simulink model "NUOVO_MODELLO_COPPIE_VELOCITA"  (R2021a)
settings: Solver=VariableStepAuto  StartTime=0.0  StopTime=3  RelTol=1e-3
values from neighbouring files (symbols this model uses):
  A = [1 Ts;0 1]    [parameters.m]
  Be = 1    [parameters.m]
  beta = 2*pi*Fc*Ts / (1+2*pi*Fc*Ts)    (= 0.00624395339097)    [parameters.m]
  Bh = 0.002    [parameters.m]
  Bh_hat = 0.0002    [parameters.m]
  C = [1 0]    [parameters.m]
  delayCommM2S = 0    [parameters.m]
  delayCommS2M = 0    [parameters.m]
  dt = 0.5    [parameters.m]
  Fc = 1    [parameters.m]
  Jh = 0.00002    (= 2e-05)    [parameters.m]
  k_m = 19.34    [parameters.m]
  k_s = 19.34    [parameters.m]
  Kc2v_m = 2    [parameters.m]
  Kc2v_s = 2    [parameters.m]
  Kd_h = 1.125    [parameters.m]
  Ke = 10    [parameters.m]
  Kh_hat = 0.0002    [parameters.m]
  Kh_max = 50    [parameters.m]
  Kp_h = 0.8    [parameters.m]
  Kt2c_m = 1.182    [parameters.m]
  Kt2c_s = 1.182    [parameters.m]
  lArm_m = 0.1    [parameters.m]
  lArm_s = 0.1    [parameters.m]
  noise_threshold = 0.05    [parameters.m]
  PosRef = 1    [parameters.m]
  qe = 2    [parameters.m]
  stopTime = str2double(stopTime)    [parameters.m]
  tau_m = 1.217    [parameters.m]
  tau_s = 1.217    [parameters.m]
  Ts = 0.001    [parameters.m]
  Variance = 0.00000001    (= 1e-08)    [parameters.m]
undefined symbols (not defined in the file or in its folder): DiscIntNeverNeededParam, Discrete, Time
libraries: simulink_extras x20, dspsigops x20, ctrlSharedLib x7, cstblocks x1
settings Model: Creator=mirko  LastModifiedBy=mirko

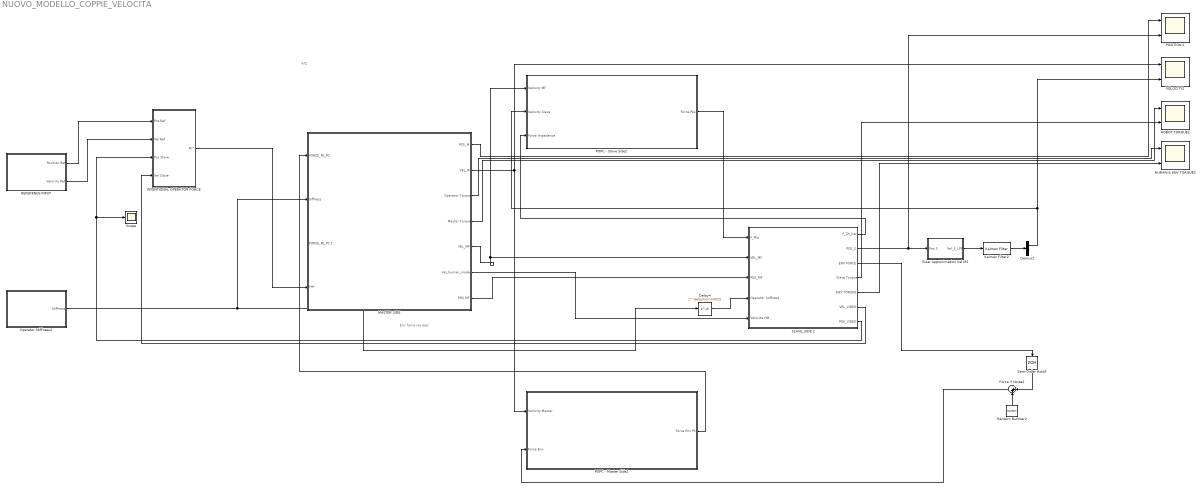
== system NUOVO_MODELLO_COPPIE_VELOCITA ==
  note: A/Z
  note: Env force revised
  Delay4 : Delay  DelayLength=delayCommM2S  SampleTime=Ts
  Demux2 : Demux  Outputs=2
  Euler Approximation Vel M2 : Subsystem
  Force + Noise2 : Sum  Inputs=|++
  HUMAN & ENV TORQUE2 : Scope  NumInputPorts=2
  INTENTIONAL OPERATOR FORCE : Subsystem
  Kalman Filter2 : ctrlSharedLib/Kalman Filter  TimeDomain=Discrete-Time  UseCurrentEstimator=off  ModelSource=Individual A, B, C, D matrices  ModelSourceVariable=ss(A,0,C,0)  A=A  B=1  C=C  D=0  NumberOfStates=2  NumberOfInputs=1  NumberOfOutputs=1  InitialEstimateSource=Dialog  X0=0  P0=10  UseK=off  UseGH=off  NumberOfProcessNoiseInputs=1  G=1  TimeInvariantG=on  H=0  TimeInvariantH=on  Q=0.05  TimeInvariantQ=on  R=1  TimeInvariantR=on  N=0  TimeInvariantN=on  AddInputPort=off  AddEnablePort=off  OutputEstimatedY=off  OutputP=off  Ts=Ts
  MASTER SIDE : Subsystem
  Operator Stiffness2 : Subsystem
  POPC - Master Side2 : Subsystem
  POPC - Slave Side2 : Subsystem
  POSITION 2 : Scope  NumInputPorts=2
  REFERENCE INPUT : Subsystem
  ROBOT TORQUE2 : Scope  NumInputPorts=2
  Random Number2 : RandomNumber  Variance=Variance  SampleTime=Ts
  SLAVE_SIDE 2 : Subsystem
  Scope : Scope
  VELOCITY2 : Scope  NumInputPorts=2
  Zero-Order Hold3 : ZeroOrderHold  SampleTime=Ts
  wires:
  Operator Stiffness2/1(Stiffness) -> Delay4/1, MASTER SIDE/2(Siffness)
  Force + Noise2/1 -> POPC - Master Side2/2(Force Env)
  REFERENCE INPUT/2("Velocity Ref ") -> INTENTIONAL OPERATOR FORCE/2(Vel Ref)
  POPC - Slave Side2/1(Force PCs) -> SLAVE_SIDE 2/1(F_PCs)
  Demux2/1 -> VELOCITY2/2, POPC - Slave Side2/2(Velocity Slave)
  SLAVE_SIDE 2/1(F_Zh_hat) -> POPC - Slave Side2/3(Force Impedence)
  MASTER SIDE/4(Master Torque) -> ROBOT TORQUE2/1
  Random Number2/1 -> Force + Noise2/2
  MASTER SIDE/3(Operator Torque) -> HUMAN & ENV TORQUE2/1
  SLAVE_SIDE 2/2(POS_S) -> POSITION 2/2, Euler Approximation Vel M2/1(Pos S)
  REFERENCE INPUT/1("Position Ref ") -> INTENTIONAL OPERATOR FORCE/1(Pos Ref)
  POPC - Master Side2/1(Force Env PC) -> MASTER SIDE/1("FORCE_FE_PC ")
  SLAVE_SIDE 2/7(POS_VIDEO) -> INTENTIONAL OPERATOR FORCE/3(Pos Slave), Scope/1
  SLAVE_SIDE 2/3(ENV FORCE) -> Zero-Order Hold3/1
  SLAVE_SIDE 2/5(ENV TORQUE) -> HUMAN & ENV TORQUE2/2
  SLAVE_SIDE 2/6(VEL_VIDEO) -> INTENTIONAL OPERATOR FORCE/4(Vel Slave)
  MASTER SIDE/2(VEL_M) -> POPC - Master Side2/1(Velocity Master), VELOCITY2/1
  Kalman Filter2/1 -> Demux2/1
  Delay4/1 -> SLAVE_SIDE 2/4(Operator Stiffness)
  Zero-Order Hold3/1 -> Force + Noise2/1
  Euler Approximation Vel M2/1("Vel_S_LPF ") -> Kalman Filter2/1
  SLAVE_SIDE 2/4(Slave Torque) -> ROBOT TORQUE2/2
  MASTER SIDE/1(POS_M) -> POSITION 2/1
  INTENTIONAL OPERATOR FORCE/1("Fh* ") -> MASTER SIDE/4(FH*)
  MASTER SIDE/5(VEL_MF) -> POPC - Slave Side2/1(Velocity MF), SLAVE_SIDE 2/2(VEL_MF)
  MASTER SIDE/6(Vel_human_model) -> SLAVE_SIDE 2/5("Velocità HM ")
  MASTER SIDE/7(POS MF) -> SLAVE_SIDE 2/3(POS_MF)

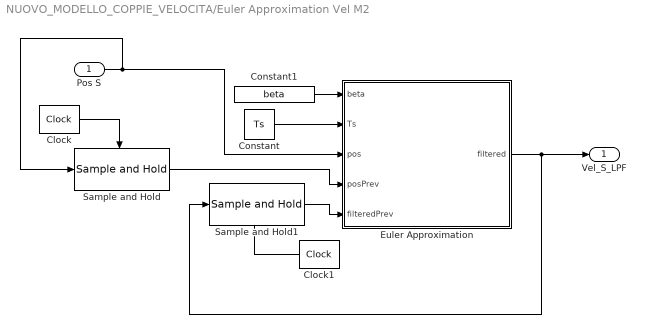
== system NUOVO_MODELLO_COPPIE_VELOCITA/Euler Approximation Vel M2 ==
  Pos S : Inport
  Clock : simulink_extras/Flip Flops/Clock  period=Ts*2
  Clock1 : simulink_extras/Flip Flops/Clock  period=Ts*2
  Constant : Constant  Value=Ts
  Constant1 : Constant  Value=beta
  "Euler Approximation " : MATLAB Function  TreatAsAtomicUnit=on
  Sample and Hold : dspsigops/Sample and Hold  trig=Rising edge  initCond=0  latchinput=on
  Sample and Hold1 : dspsigops/Sample and Hold  trig=Rising edge  initCond=0  latchinput=on
  "Vel_S_LPF " : Outport
  wires:
  Pos S/1 -> Sample and Hold/1, "Euler Approximation "/3(pos)
  Constant/1 -> "Euler Approximation "/2(Ts)
  Sample and Hold/1 -> "Euler Approximation "/4(posPrev)
  Clock/1 -> Sample and Hold/Trigger
  Sample and Hold1/1 -> "Euler Approximation "/5(filteredPrev)
  "Euler Approximation "/1(filtered) -> "Vel_S_LPF "/1, Sample and Hold1/1
  Clock1/1 -> Sample and Hold1/Trigger
  Constant1/1 -> "Euler Approximation "/1(beta)

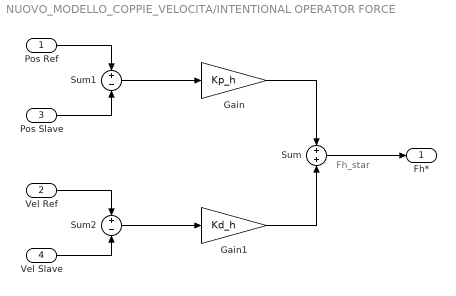
== system NUOVO_MODELLO_COPPIE_VELOCITA/INTENTIONAL OPERATOR FORCE ==
  note: Fh_star
  Pos Ref : Inport
  Vel Ref : Inport  Port=2
  Pos Slave : Inport  Port=3
  Vel Slave : Inport  Port=4
  Gain : Gain  Gain=Kp_h
  Gain1 : Gain  Gain=Kd_h
  Sum : Sum
  Sum1 : Sum  Inputs=+-
  Sum2 : Sum  Inputs=+-
  "Fh* " : Outport
  wires:
  Pos Ref/1 -> Sum1/1
  Pos Slave/1 -> Sum1/2
  Vel Ref/1 -> Sum2/1
  Vel Slave/1 -> Sum2/2
  Sum1/1 -> Gain/1
  Sum2/1 -> Gain1/1
  Gain1/1 -> Sum/2
  Gain/1 -> Sum/1
  Sum/1 -> "Fh* "/1

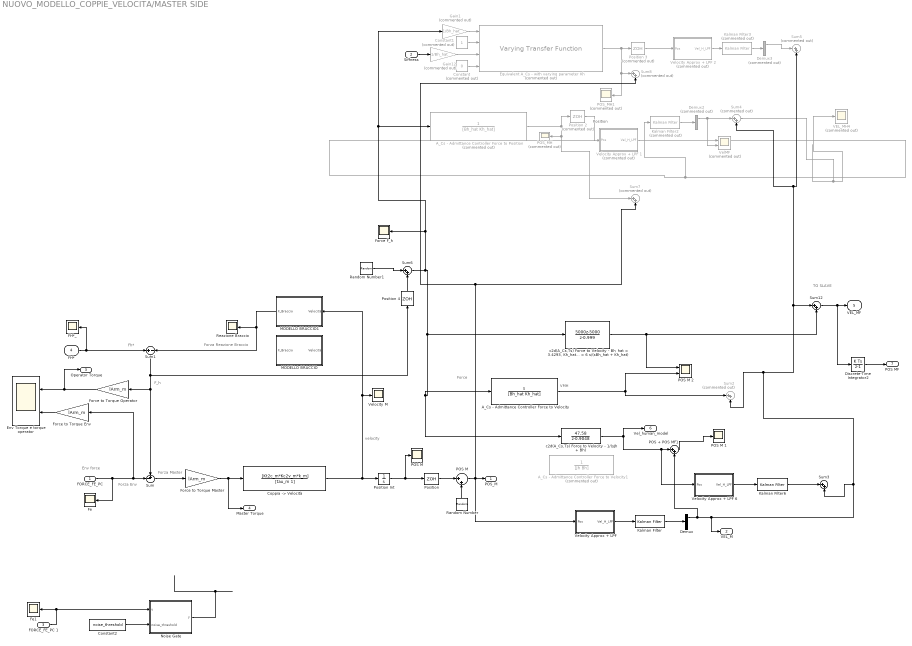
== system NUOVO_MODELLO_COPPIE_VELOCITA/MASTER SIDE ==
  note: Forza Master
  note: VMH
  note: Position
  note: Env force
  note: Force
  note: F_h
  note: Forza Reazione Braccio
  note: Fh*
  note: velocity
  note: TO SLAVE
  note: Forza Env
  "FORCE_FE_PC " : Inport
  Siffness : Inport  Port=2
  FORCE_FE_PC 1 : Inport  Port=3
  FH* : Inport  Port=4
  A_Cs - Admittance Controller Force to Position : TransferFcn  Commented=on  Denominator=[Bh_hat Kh_hat]
  A_Cs - Admittance Controller Force to Velocity : TransferFcn  Numerator=[1 0]  Denominator=[Bh_hat Kh_hat]
  A_Cs - Admittance Controller Force to Velocity1 : TransferFcn  Commented=on  Denominator=[Jh Bh]
  Constant : Constant  Commented=on  Value=0
  Constant1 : Constant  Commented=on
  Constant2 : Constant  Value=noise_threshold
  "Coppia -> Velocità" : TransferFcn  Numerator=[Kt2c_m*Kc2v_m*k_m]  Denominator=[tau_m 1]
  Demux : Demux  Outputs=2
  Demux2 : Demux  Commented=on  Outputs=2
  Demux3 : Demux  Commented=on  Outputs=2
  Discrete-Time Integrator2 : DiscreteIntegrator  SampleTime=-1  ICPrevOutput=DiscIntNeverNeededParam  ICPrevScaledInput=DiscIntNeverNeededParam
  "Env Torque e torque operator " : Scope  NumInputPorts=2
  Equivalent A_Cs - with varying parameter Kh : cstblocks/Linear Parameter Varying/Varying Transfer Function  Commented=on  N=1
  FH*_ : Scope
  Fe : Scope
  Fe1 : Scope
  "Force F_h " : Scope
  Force to Torque Env : Gain  Gain=lArm_m
  Force to Torque Master : Gain  Gain=lArm_m
  Force to Torque Operator : Gain  Gain=lArm_m
  Gain1 : Gain  Commented=on  Gain=1/Bh_hat
  Gain12 : Gain  Commented=on  Gain=1/Bh_hat
  Kalman Filter : ctrlSharedLib/Kalman Filter  TimeDomain=Discrete-Time  UseCurrentEstimator=off  ModelSource=Individual A, B, C, D matrices  ModelSourceVariable=ss(A,0,C,0)  A=A  B=1  C=C  D=0  NumberOfStates=2  NumberOfInputs=1  NumberOfOutputs=1  InitialEstimateSource=Dialog  X0=0  P0=10  UseK=off  UseGH=off  NumberOfProcessNoiseInputs=1  G=1  TimeInvariantG=on  H=0  TimeInvariantH=on  Q=0.05  TimeInvariantQ=on  R=1  TimeInvariantR=on  N=0  TimeInvariantN=on  AddInputPort=off  AddEnablePort=off  OutputEstimatedY=off  OutputP=off  Ts=Ts
  Kalman Filter2 : ctrlSharedLib/Kalman Filter  Commented=on  TimeDomain=Discrete-Time  UseCurrentEstimator=off  ModelSource=Individual A, B, C, D matrices  ModelSourceVariable=ss(A,0,C,0)  A=A  B=1  C=C  D=0  NumberOfStates=2  NumberOfInputs=1  NumberOfOutputs=1  InitialEstimateSource=Dialog  X0=0  P0=10  UseK=off  UseGH=off  NumberOfProcessNoiseInputs=1  G=1  TimeInvariantG=on  H=0  TimeInvariantH=on  Q=0.05  TimeInvariantQ=on  R=1  TimeInvariantR=on  N=0  TimeInvariantN=on  AddInputPort=off  AddEnablePort=off  OutputEstimatedY=off  OutputP=off  Ts=Ts
  Kalman Filter3 : ctrlSharedLib/Kalman Filter  Commented=on  TimeDomain=Discrete-Time  UseCurrentEstimator=off  ModelSource=Individual A, B, C, D matrices  ModelSourceVariable=ss(A,0,C,0)  A=A  B=1  C=C  D=0  NumberOfStates=2  NumberOfInputs=1  NumberOfOutputs=1  InitialEstimateSource=Dialog  X0=0  P0=10  UseK=off  UseGH=off  NumberOfProcessNoiseInputs=1  G=1  TimeInvariantG=on  H=0  TimeInvariantH=on  Q=0.05  TimeInvariantQ=on  R=1  TimeInvariantR=on  N=0  TimeInvariantN=on  AddInputPort=off  AddEnablePort=off  OutputEstimatedY=off  OutputP=off  Ts=Ts
  Kalman Filter6 : ctrlSharedLib/Kalman Filter  TimeDomain=Discrete-Time  UseCurrentEstimator=off  ModelSource=Individual A, B, C, D matrices  ModelSourceVariable=ss(A,0,C,0)  A=A  B=1  C=C  D=0  NumberOfStates=2  NumberOfInputs=1  NumberOfOutputs=1  InitialEstimateSource=Dialog  X0=0  P0=10  UseK=off  UseGH=off  NumberOfProcessNoiseInputs=1  G=1  TimeInvariantG=on  H=0  TimeInvariantH=on  Q=0.05  TimeInvariantQ=on  R=1  TimeInvariantR=on  N=0  TimeInvariantN=on  AddInputPort=off  AddEnablePort=off  OutputEstimatedY=off  OutputP=off  Ts=Ts
  MODELLO BRACCIO : Subsystem
  MODELLO BRACCIO1 : Subsystem
  Noise Gate : MATLAB Function  TreatAsAtomicUnit=on
  POS + POS MF1 : Sum  Inputs=|++
  POS M : Sum  Inputs=|++
  "POS M " : Scope
  POS M 1 : Scope
  POS M 2 : Scope  NumInputPorts=2
  POS_MH : Scope  Commented=on
  POS_MH1 : Scope  Commented=on
  "Position " : ZeroOrderHold  SampleTime=Ts
  Position 2 : ZeroOrderHold  Commented=on  SampleTime=Ts
  Position 3 : ZeroOrderHold  Commented=on  SampleTime=Ts
  Position 4 : ZeroOrderHold  SampleTime=Ts
  "Position Int " : Integrator
  Random Number : RandomNumber  Variance=Variance  SampleTime=Ts
  Random Number1 : RandomNumber  Variance=Variance  SampleTime=Ts
  Reazione Braccio : Scope
  Sum : Sum  Inputs=+-|
  Sum1 : Sum  Inputs=+-
  Sum12 : Sum  Inputs=|++
  Sum{2,4..5,7..8} (5 alike) : Sum  Commented=on  Inputs=|++
  Sum3 : Sum  Inputs=|++
  Sum6 : Sum  Inputs=|++
  VEL_MH4 : Scope  Commented=on
  VelMF : Scope  Commented=on  NumInputPorts=2
  "Velocity Approx + LPF " : Subsystem
  Velocity Approx + LPF 1 : Subsystem  Commented=on
  Velocity Approx + LPF 2 : Subsystem  Commented=on
  Velocity Approx + LPF 6 : Subsystem
  Velocity M : Scope
  c2d(A_Cs,Ts) Force to Velocity - 1/(sJh + Bh) : DiscreteTransferFcn  Numerator=[47.58]  Denominator=[1 -0.9048]  SampleTime=Ts
  "c2d(A_Cs,Ts) Force to Velocity - Bh_hat = 3.4293, Kh_hat = 6 s/(sBh_hat + Kh_hat)" : DiscreteTransferFcn  Numerator=[5000 -5000]  Denominator=[1 -0.999]  SampleTime=Ts
  POS_M : Outport
  VEL_M : Outport  Port=2
  Operator Torque : Outport  Port=3
  Master Torque : Outport  Port=4
  VEL_MF : Outport  Port=5
  Vel_human_model : Outport  Port=6
  POS MF : Outport  Port=7
  wires:
  "Position Int "/1 -> "Position "/1, "POS M "/1
  "Coppia -> Velocità"/1 -> "Position Int "/1, MODELLO BRACCIO1/1("Velocità "), Velocity M/1
  Force to Torque Operator/1 -> "Env Torque e torque operator "/1, Operator Torque/1
  MODELLO BRACCIO1/1(F_Braccio) -> Sum1/2, Reazione Braccio/1
  "FORCE_FE_PC "/1 -> Force to Torque Env/1, Sum/2, Fe/1
  FH*/1 -> Sum1/1, FH*_/1
  Constant/1 -> Equivalent A_Cs - with varying parameter Kh/4
  Gain12/1 -> Equivalent A_Cs - with varying parameter Kh/3
  Siffness/1 -> Gain12/1
  Constant1/1 -> Equivalent A_Cs - with varying parameter Kh/2
  Equivalent A_Cs - with varying parameter Kh/1 -> Position 3/1, POS_MH1/1, Sum8/1
  A_Cs - Admittance Controller Force to Position/1 -> Position 2/1, Sum7/1, POS_MH/1
  Sum4/1 -> VEL_MH4/1
  Gain1/1 -> Equivalent A_Cs - with varying parameter Kh/1
  Velocity Approx + LPF 1/1("Vel_H_LPF ") -> VelMF/1, Kalman Filter2/1
  Velocity Approx + LPF 2/1("Vel_H_LPF ") -> Kalman Filter3/1
  Random Number/1 -> POS M/2
  POS M/1 -> "Velocity Approx + LPF "/1(Pos), Sum7/2, Sum8/2, POS_M/1
  "Velocity Approx + LPF "/1("Vel_H_LPF ") -> Kalman Filter/1
  "Position "/1 -> POS M/1
  Demux/1 -> POS + POS MF1/2, Sum3/2, Sum4/2, Sum5/2, Sum12/1, Sum2/2, VEL_M/1
  Kalman Filter/1 -> Demux/1
  A_Cs - Admittance Controller Force to Velocity/1 -> Sum2/1, POS M 2/2
  Demux2/1 -> VelMF/2, Sum4/1
  Kalman Filter2/1 -> Demux2/1
  Position 2/1 -> Velocity Approx + LPF 1/1(Pos)
  Position 3/1 -> Velocity Approx + LPF 2/1(Pos)
  Demux3/1 -> Sum5/1
  Kalman Filter3/1 -> Demux3/1
  Sum/1 -> Force to Torque Master/1
  Random Number1/1 -> Sum6/1
  Sum6/1 -> c2d(A_Cs,Ts) Force to Velocity - 1/(sJh + Bh)/1, A_Cs - Admittance Controller Force to Velocity/1, "c2d(A_Cs,Ts) Force to Velocity - Bh_hat = 3.4293, Kh_hat = 6 s/(sBh_hat + Kh_hat)"/1, Gain1/1, A_Cs - Admittance Controller Force to Position/1, "Force F_h "/1
  Constant2/1 -> Noise Gate/2(noise_threshold)
  Noise Gate/1(y) -> ?
  FORCE_FE_PC 1/1 -> Noise Gate/1(u), Fe1/1
  Force to Torque Env/1 -> "Env Torque e torque operator "/2
  Force to Torque Master/1 -> "Coppia -> Velocità"/1, Master Torque/1
  Sum1/1 -> Position 4/1, Sum/1, Force to Torque Operator/1
  Position 4/1 -> Sum6/2
  "c2d(A_Cs,Ts) Force to Velocity - Bh_hat = 3.4293, Kh_hat = 6 s/(sBh_hat + Kh_hat)"/1 -> POS M 2/1, Sum12/2
  Sum12/1 -> Discrete-Time Integrator2/1, VEL_MF/1
  POS + POS MF1/1 -> POS M 1/1
  Velocity Approx + LPF 6/1("Vel_H_LPF ") -> Kalman Filter6/1
  Kalman Filter6/1 -> Sum3/1
  c2d(A_Cs,Ts) Force to Velocity - 1/(sJh + Bh)/1 -> Velocity Approx + LPF 6/1(Pos), POS + POS MF1/1, Vel_human_model/1
  Discrete-Time Integrator2/1 -> POS MF/1

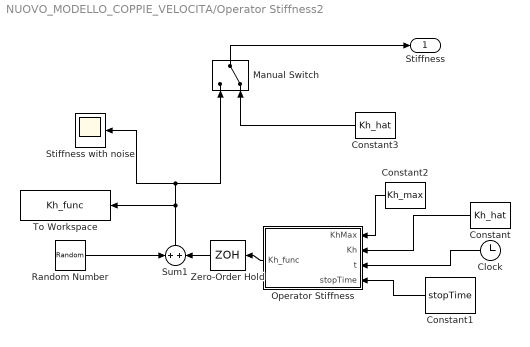
== system NUOVO_MODELLO_COPPIE_VELOCITA/Operator Stiffness2 ==
  Clock : Clock
  Constant : Constant  Value=Kh_hat
  Constant1 : Constant  Value=stopTime  SampleTime=Ts
  Constant2 : Constant  Value=Kh_max
  Constant3 : Constant  Value=Kh_hat
  Manual Switch : ManualSwitch  CurrentSetting=0
  "Operator Stiffness " : MATLAB Function  TreatAsAtomicUnit=on
  Random Number : RandomNumber  Variance=Variance  SampleTime=Ts
  Stiffness with noise : Scope
  Sum1 : Sum
  To Workspace : ToWorkspace  VariableName=Kh_func  SaveFormat=Structure With Time  SampleTime=-1
      settings: Save2DSignal=2-D array (concatenate along first dimension)
  Zero-Order Hold : ZeroOrderHold  SampleTime=-1
  Stiffness : Outport
  wires:
  Constant3/1 -> Manual Switch/2
  Sum1/1 -> To Workspace/1, Manual Switch/1, Stiffness with noise/1
  Constant2/1 -> "Operator Stiffness "/1(KhMax)
  "Operator Stiffness "/1(Kh_func) -> Zero-Order Hold/1
  Clock/1 -> "Operator Stiffness "/3(t)
  Random Number/1 -> Sum1/1
  Constant/1 -> "Operator Stiffness "/2(Kh)
  Constant1/1 -> "Operator Stiffness "/4(stopTime)
  Manual Switch/1 -> Stiffness/1
  Zero-Order Hold/1 -> Sum1/2

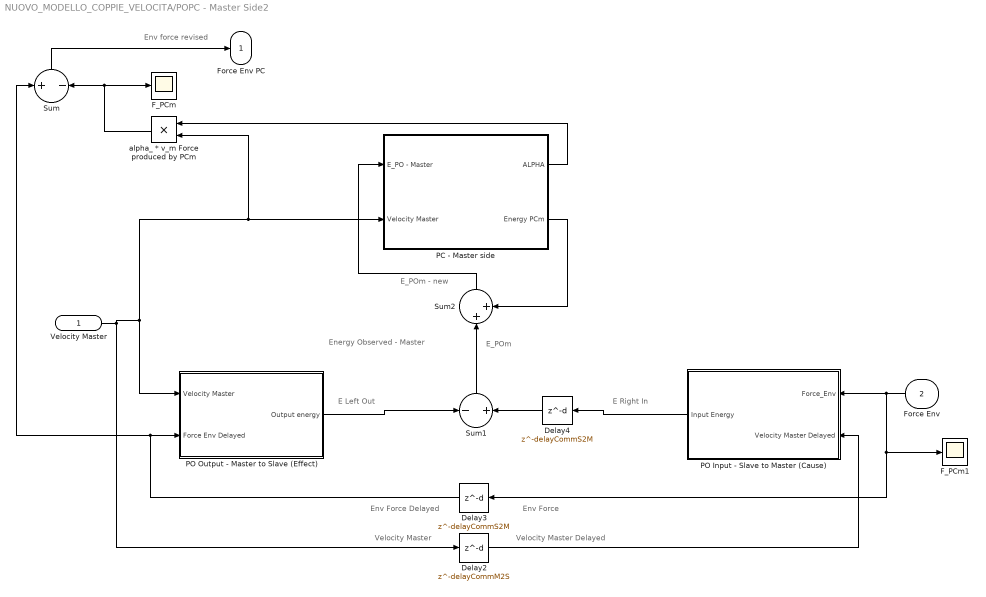
== system NUOVO_MODELLO_COPPIE_VELOCITA/POPC - Master Side2 ==
  note: E_POm
  note: Energy Observed - Master
  note: Env force revised
  note: Env Force Delayed
  note: Env Force
  note: Velocity Master
  note: Velocity Master Delayed
  note: E Left Out
  note: E Right In
  note: E_POm - new
  Velocity Master : Inport
  Force Env : Inport  Port=2
  Delay2 : Delay  DelayLength=delayCommM2S  InitialCondition=0  SampleTime=Ts
  Delay3 : Delay  DelayLength=delayCommS2M  InitialCondition=0  SampleTime=Ts
  Delay4 : Delay  DelayLength=delayCommS2M  InitialCondition=0
  F_PCm : Scope
  F_PCm1 : Scope
  PC - Master side : Subsystem
  PO Input - Slave to Master (Cause) : Subsystem
  PO Output - Master to Slave (Effect) : Subsystem
  Sum : Sum  Inputs=+-
  Sum1 : Sum  Inputs=-+
  Sum2 : Sum  Inputs=|++
  alpha_ * v_m Force produced by PCm : Product
  Force Env PC : Outport
  wires:
  alpha_ * v_m Force produced by PCm/1 -> Sum/2, F_PCm/1
  Force Env/1 -> Delay3/1, F_PCm1/1, PO Input - Slave to Master (Cause)/1(Force_Env)
  Delay3/1 -> Sum/1, PO Output - Master to Slave (Effect)/2(Force Env Delayed)
  Velocity Master/1 -> Delay2/1, alpha_ * v_m Force produced by PCm/2, PC - Master side/2("Velocity Master "), PO Output - Master to Slave (Effect)/1(Velocity Master)
  Sum1/1 -> Sum2/1
  Sum/1 -> Force Env PC/1
  PO Output - Master to Slave (Effect)/1(Output energy) -> Sum1/1
  Delay4/1 -> Sum1/2
  Delay2/1 -> PO Input - Slave to Master (Cause)/2(Velocity Master Delayed)
  PO Input - Slave to Master (Cause)/1(Input Energy) -> Delay4/1
  Sum2/1 -> PC - Master side/1(E_PO - Master)
  PC - Master side/1(ALPHA) -> alpha_ * v_m Force produced by PCm/1
  PC - Master side/2(Energy PCm) -> Sum2/2

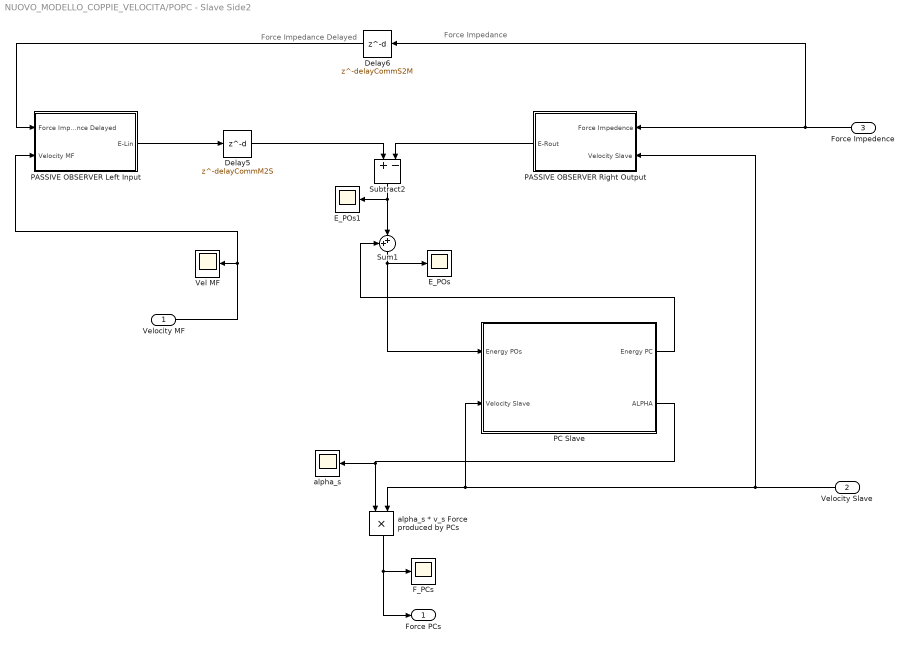
== system NUOVO_MODELLO_COPPIE_VELOCITA/POPC - Slave Side2 ==
  note: Force Impedance Delayed
  note: Force Impedance
  Velocity MF : Inport
  Velocity Slave : Inport  Port=2
  Force Impedence : Inport  Port=3
  Delay5 : Delay  DelayLength=delayCommM2S  InitialCondition=0  SampleTime=Ts
  Delay6 : Delay  DelayLength=delayCommS2M  InitialCondition=0  SampleTime=Ts
  E_POs : Scope
  E_POs1 : Scope
  F_PCs : Scope
  PASSIVE OBSERVER Left Input : Subsystem
  PASSIVE OBSERVER Right Output : Subsystem
  PC Slave : Subsystem
  Subtract2 : Sum  Inputs=+|-
  Sum1 : Sum  Inputs=++|
  Vel MF : Scope
  alpha_s : Scope
  alpha_s * v_s Force produced by PCs : Product
  Force PCs : Outport
  wires:
  Subtract2/1 -> E_POs1/1, Sum1/2
  Delay6/1 -> PASSIVE OBSERVER Left Input/1(Force Impedance Delayed)
  Velocity Slave/1 -> PASSIVE OBSERVER Right Output/2(Velocity Slave), alpha_s * v_s Force produced by PCs/2, PC Slave/2(Velocity Slave)
  Sum1/1 -> PC Slave/1(Energy POs), E_POs/1
  Delay5/1 -> Subtract2/1
  alpha_s * v_s Force produced by PCs/1 -> Force PCs/1, F_PCs/1
  PASSIVE OBSERVER Left Input/1(E-Lin) -> Delay5/1
  Velocity MF/1 -> PASSIVE OBSERVER Left Input/2(Velocity MF), Vel MF/1
  PASSIVE OBSERVER Right Output/1(E-Rout) -> Subtract2/2
  Force Impedence/1 -> Delay6/1, PASSIVE OBSERVER Right Output/1(Force Impedence)
  PC Slave/2(ALPHA) -> alpha_s * v_s Force produced by PCs/1, alpha_s/1
  PC Slave/1(Energy PC) -> Sum1/1

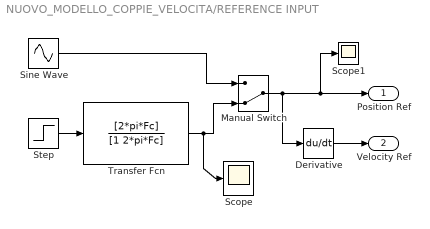
== system NUOVO_MODELLO_COPPIE_VELOCITA/REFERENCE INPUT ==
  Derivative : Derivative
  Manual Switch : ManualSwitch  CurrentSetting=0
  Scope : Scope
  Scope1 : Scope
  Sine Wave : Sin  Amplitude=PosRef  SampleTime=0
  Step : Step  Time=0.5  After=PosRef  SampleTime=0
  Transfer Fcn : TransferFcn  Numerator=[2*pi*Fc]  Denominator=[1 2*pi*Fc]
  "Position Ref " : Outport
  "Velocity Ref " : Outport  Port=2
  wires:
  Sine Wave/1 -> Manual Switch/1
  Derivative/1 -> "Velocity Ref "/1
  Manual Switch/1 -> Derivative/1, Scope1/1, "Position Ref "/1
  Transfer Fcn/1 -> Scope/1, Manual Switch/2
  Step/1 -> Transfer Fcn/1

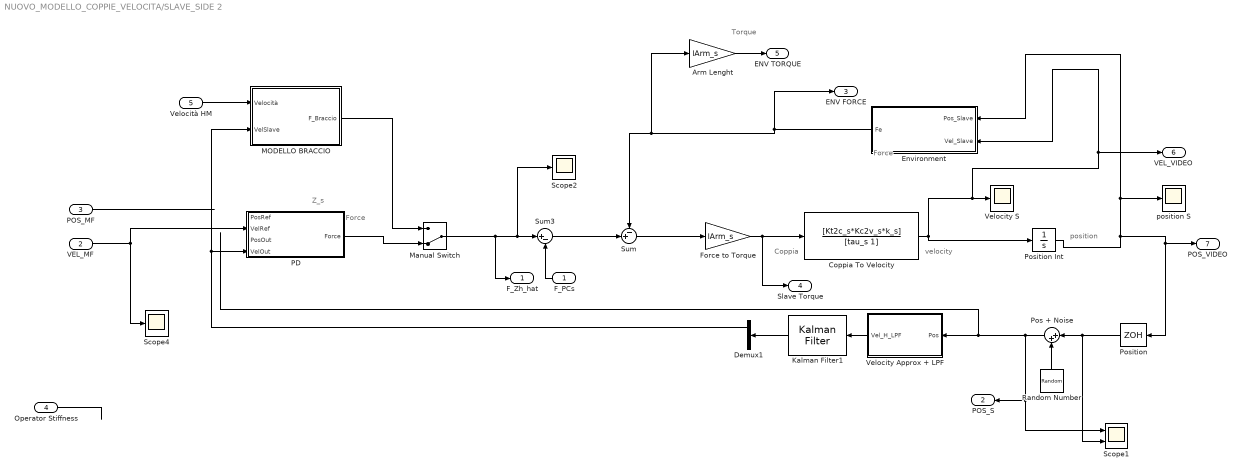
== system NUOVO_MODELLO_COPPIE_VELOCITA/SLAVE_SIDE 2 ==
  note: Force
  note: velocity
  note: position
  note: Coppia
  note: Torque
  note: Z_s
  note: Force
  F_PCs : Inport
  VEL_MF : Inport  Port=2
  POS_MF : Inport  Port=3
  Operator Stiffness : Inport  Port=4
  "Velocità HM " : Inport  Port=5
  Arm Lenght : Gain  Gain=lArm_s
  "Coppia To Velocity " : TransferFcn  Numerator=[Kt2c_s*Kc2v_s*k_s]  Denominator=[tau_s 1]
  Demux1 : Demux  Outputs=2
  "Environment " : Subsystem
  Force to Torque : Gain  Gain=lArm_s
  Kalman Filter1 : ctrlSharedLib/Kalman Filter  TimeDomain=Discrete-Time  UseCurrentEstimator=off  ModelSource=Individual A, B, C, D matrices  ModelSourceVariable=ss(A,0,C,0)  A=A  B=1  C=C  D=0  NumberOfStates=2  NumberOfInputs=1  NumberOfOutputs=1  InitialEstimateSource=Dialog  X0=0  P0=10  UseK=off  UseGH=off  NumberOfProcessNoiseInputs=1  G=1  TimeInvariantG=on  H=0  TimeInvariantH=on  Q=0.05  TimeInvariantQ=on  R=1  TimeInvariantR=on  N=0  TimeInvariantN=on  AddInputPort=off  AddEnablePort=off  OutputEstimatedY=off  OutputP=off  Ts=Ts
  MODELLO BRACCIO : Subsystem
  Manual Switch : ManualSwitch  CurrentSetting=0
  PD : Subsystem
  Pos + Noise : Sum  Inputs=|++
  Position : ZeroOrderHold  SampleTime=Ts
  "Position Int " : Integrator
  Random Number : RandomNumber  Variance=Variance  SampleTime=Ts
  Scope1 : Scope  NumInputPorts=2
  Scope2 : Scope
  Scope4 : Scope
  Sum : Sum  Inputs=-+|
  Sum3 : Sum  Inputs=|+-
  "Velocity Approx + LPF " : Subsystem
  Velocity S : Scope
  "position S " : Scope
  F_Zh_hat : Outport
  POS_S : Outport  Port=2
  ENV FORCE : Outport  Port=3
  Slave Torque : Outport  Port=4
  ENV TORQUE : Outport  Port=5
  VEL_VIDEO : Outport  Port=6
  POS_VIDEO : Outport  Port=7
  wires:
  "Position Int "/1 -> Position/1, POS_VIDEO/1, "position S "/1, "Environment "/1(Pos_Slave)
  "Environment "/1(Fe) -> Sum/1, Arm Lenght/1, ENV FORCE/1
  "Coppia To Velocity "/1 -> "Position Int "/1, "Environment "/2("Vel_Slave "), VEL_VIDEO/1, Velocity S/1
  Manual Switch/1 -> Scope2/1, Sum3/1, F_Zh_hat/1
  Sum3/1 -> Sum/2
  F_PCs/1 -> Sum3/2
  Operator Stiffness/1 -> ?
  VEL_MF/1 -> Scope4/1, PD/2(VelRef)
  Pos + Noise/1 -> "Velocity Approx + LPF "/1(Pos), POS_S/1, Scope1/1
  Random Number/1 -> Pos + Noise/2
  Demux1/1 -> MODELLO BRACCIO/2(VelSlave), PD/4(VelOut)
  Position/1 -> Scope1/2, Pos + Noise/1
  "Velocity Approx + LPF "/1("Vel_H_LPF ") -> Kalman Filter1/1
  Kalman Filter1/1 -> Demux1/1
  Sum/1 -> Force to Torque/1
  POS_MF/1 -> ?
  Force to Torque/1 -> Slave Torque/1, "Coppia To Velocity "/1
  Arm Lenght/1 -> ENV TORQUE/1
  "Velocità HM "/1 -> MODELLO BRACCIO/1("Velocità ")
  MODELLO BRACCIO/1(F_Braccio) -> Manual Switch/1
  PD/1(Force) -> Manual Switch/2

== system NUOVO_MODELLO_COPPIE_VELOCITA/MASTER SIDE/MODELLO BRACCIO ==
  "Velocità " : Inport
  Derivative : Derivative  CoefficientInTFapproximation=0.01
  Friction : Gain  Gain=Bh
  Inertia : Gain  Gain=Jh
  Sum : Sum  Inputs=+++
  F_Braccio : Outport
  wires:
  "Velocità "/1 -> Friction/1, Derivative/1
  Derivative/1 -> Inertia/1
  Inertia/1 -> Sum/2
  Friction/1 -> Sum/1
  Sum/1 -> F_Braccio/1

== system NUOVO_MODELLO_COPPIE_VELOCITA/MASTER SIDE/MODELLO BRACCIO1 ==
  "Velocità " : Inport
  Friction : Gain  Gain=Kh_hat
  Friction1 : Gain  Gain=Bh_hat
  Integrator : Integrator
  Sum : Sum  Inputs=+++
  F_Braccio : Outport
  wires:
  Sum/1 -> F_Braccio/1
  Friction/1 -> Sum/1
  Friction1/1 -> Sum/2
  "Velocità "/1 -> Integrator/1, Friction1/1
  Integrator/1 -> Friction/1

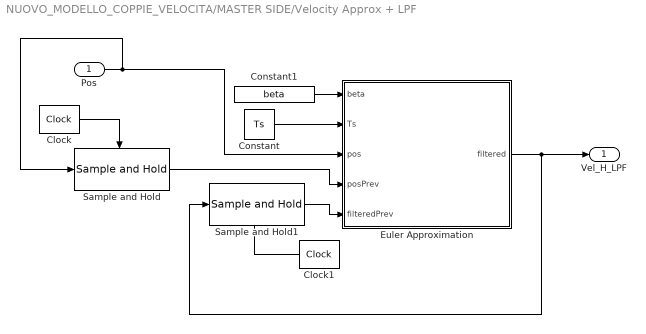
== system NUOVO_MODELLO_COPPIE_VELOCITA/MASTER SIDE/Velocity Approx + LPF  ==
  Pos : Inport
  Clock : simulink_extras/Flip Flops/Clock  period=Ts*2
  Clock1 : simulink_extras/Flip Flops/Clock  period=Ts*2
  Constant : Constant  Value=Ts
  Constant1 : Constant  Value=beta
  "Euler Approximation " : MATLAB Function  TreatAsAtomicUnit=on
  Sample and Hold : dspsigops/Sample and Hold  trig=Rising edge  initCond=0  latchinput=on
  Sample and Hold1 : dspsigops/Sample and Hold  trig=Rising edge  initCond=0  latchinput=on
  "Vel_H_LPF " : Outport
  wires:
  Pos/1 -> Sample and Hold/1, "Euler Approximation "/3(pos)
  Constant/1 -> "Euler Approximation "/2(Ts)
  Sample and Hold/1 -> "Euler Approximation "/4(posPrev)
  Clock/1 -> Sample and Hold/Trigger
  Sample and Hold1/1 -> "Euler Approximation "/5(filteredPrev)
  "Euler Approximation "/1(filtered) -> "Vel_H_LPF "/1, Sample and Hold1/1
  Clock1/1 -> Sample and Hold1/Trigger
  Constant1/1 -> "Euler Approximation "/1(beta)

== system NUOVO_MODELLO_COPPIE_VELOCITA/MASTER SIDE/Velocity Approx + LPF 1 ==
  Pos : Inport
  Clock : simulink_extras/Flip Flops/Clock  period=Ts*2
  Clock1 : simulink_extras/Flip Flops/Clock  period=Ts*2
  Constant : Constant  Value=Ts
  Constant1 : Constant  Value=beta
  "Euler Approximation " : MATLAB Function  TreatAsAtomicUnit=on
  Sample and Hold : dspsigops/Sample and Hold  trig=Rising edge  initCond=0  latchinput=on
  Sample and Hold1 : dspsigops/Sample and Hold  trig=Rising edge  initCond=0  latchinput=on
  "Vel_H_LPF " : Outport
  wires:
  Pos/1 -> Sample and Hold/1, "Euler Approximation "/3(pos)
  Constant/1 -> "Euler Approximation "/2(Ts)
  Sample and Hold/1 -> "Euler Approximation "/4(posPrev)
  Clock/1 -> Sample and Hold/Trigger
  Sample and Hold1/1 -> "Euler Approximation "/5(filteredPrev)
  "Euler Approximation "/1(filtered) -> "Vel_H_LPF "/1, Sample and Hold1/1
  Clock1/1 -> Sample and Hold1/Trigger
  Constant1/1 -> "Euler Approximation "/1(beta)

== system NUOVO_MODELLO_COPPIE_VELOCITA/MASTER SIDE/Velocity Approx + LPF 2 ==
  Pos : Inport
  Clock : simulink_extras/Flip Flops/Clock  period=Ts*2
  Clock1 : simulink_extras/Flip Flops/Clock  period=Ts*2
  Constant : Constant  Value=Ts
  Constant1 : Constant  Value=beta
  "Euler Approximation " : MATLAB Function  TreatAsAtomicUnit=on
  Sample and Hold : dspsigops/Sample and Hold  trig=Rising edge  initCond=0  latchinput=on
  Sample and Hold1 : dspsigops/Sample and Hold  trig=Rising edge  initCond=0  latchinput=on
  "Vel_H_LPF " : Outport
  wires:
  Pos/1 -> Sample and Hold/1, "Euler Approximation "/3(pos)
  Constant/1 -> "Euler Approximation "/2(Ts)
  Sample and Hold/1 -> "Euler Approximation "/4(posPrev)
  Clock/1 -> Sample and Hold/Trigger
  Sample and Hold1/1 -> "Euler Approximation "/5(filteredPrev)
  "Euler Approximation "/1(filtered) -> "Vel_H_LPF "/1, Sample and Hold1/1
  Clock1/1 -> Sample and Hold1/Trigger
  Constant1/1 -> "Euler Approximation "/1(beta)

== system NUOVO_MODELLO_COPPIE_VELOCITA/MASTER SIDE/Velocity Approx + LPF 6 ==
  Pos : Inport
  Clock : simulink_extras/Flip Flops/Clock  period=Ts*2
  Clock1 : simulink_extras/Flip Flops/Clock  period=Ts*2
  Constant : Constant  Value=Ts
  Constant1 : Constant  Value=beta
  "Euler Approximation " : MATLAB Function  TreatAsAtomicUnit=on
  Sample and Hold : dspsigops/Sample and Hold  trig=Rising edge  initCond=0  latchinput=on
  Sample and Hold1 : dspsigops/Sample and Hold  trig=Rising edge  initCond=0  latchinput=on
  "Vel_H_LPF " : Outport
  wires:
  Pos/1 -> Sample and Hold/1, "Euler Approximation "/3(pos)
  Constant/1 -> "Euler Approximation "/2(Ts)
  Sample and Hold/1 -> "Euler Approximation "/4(posPrev)
  Clock/1 -> Sample and Hold/Trigger
  Sample and Hold1/1 -> "Euler Approximation "/5(filteredPrev)
  "Euler Approximation "/1(filtered) -> "Vel_H_LPF "/1, Sample and Hold1/1
  Clock1/1 -> Sample and Hold1/Trigger
  Constant1/1 -> "Euler Approximation "/1(beta)

== system NUOVO_MODELLO_COPPIE_VELOCITA/POPC - Master Side2/PC - Master side ==
  E_PO - Master : Inport
  "Velocity Master " : Inport  Port=2
  Clock : simulink_extras/Flip Flops/Clock  period=Ts*2
  E_POm : Scope
  PASSIVE CONTROLLER PCm : MATLAB Function  TreatAsAtomicUnit=on
  Sample and Hold : dspsigops/Sample and Hold  trig=Rising edge  initCond=0  latchinput=on
  dt : Constant  Value=dt
  ALPHA : Outport
  Energy PCm : Outport  Port=2
  wires:
  Sample and Hold/1 -> PASSIVE CONTROLLER PCm/4(E_PCm_prev)
  dt/1 -> PASSIVE CONTROLLER PCm/2(dt)
  E_PO - Master/1 -> E_POm/1, PASSIVE CONTROLLER PCm/1(E_POm)
  Clock/1 -> Sample and Hold/Trigger
  PASSIVE CONTROLLER PCm/1(E_PCm) -> Sample and Hold/1, Energy PCm/1
  PASSIVE CONTROLLER PCm/2(alpha_m) -> ALPHA/1
  "Velocity Master "/1 -> PASSIVE CONTROLLER PCm/3(v_m)

== system NUOVO_MODELLO_COPPIE_VELOCITA/POPC - Master Side2/PO Input - Slave to Master (Cause) ==
  Force_Env : Inport
  Velocity Master Delayed : Inport  Port=2
  E_Rin : Scope
  PASSIVE OBSERVER S2M E Right INPUT : Subsystem
  Input Energy : Outport
  wires:
  PASSIVE OBSERVER S2M E Right INPUT/1(E-Rin) -> Input Energy/1, E_Rin/1
  Velocity Master Delayed/1 -> PASSIVE OBSERVER S2M E Right INPUT/2("Vel_M ")
  Force_Env/1 -> PASSIVE OBSERVER S2M E Right INPUT/1(Env_Force)

== system NUOVO_MODELLO_COPPIE_VELOCITA/POPC - Master Side2/PO Output - Master to Slave (Effect) ==
  note: E Left Out
  Velocity Master : Inport
  Force Env Delayed : Inport  Port=2
  E_Lout : Scope
  PASSIVE OBSERVER M2S E Left OUTPUT : Subsystem
  Output energy : Outport
  wires:
  Velocity Master/1 -> PASSIVE OBSERVER M2S E Left OUTPUT/1(Velocity Master)
  PASSIVE OBSERVER M2S E Left OUTPUT/1(E-Lout) -> Output energy/1, E_Lout/1
  Force Env Delayed/1 -> PASSIVE OBSERVER M2S E Left OUTPUT/2(Force Env Delayed)

== system NUOVO_MODELLO_COPPIE_VELOCITA/POPC - Slave Side2/PASSIVE OBSERVER Left Input ==
  Force Impedance Delayed : Inport
  Velocity MF : Inport  Port=2
  Add : Sum
  Clock : simulink_extras/Flip Flops/Clock  period=Ts*2
  Product : Product
  Sample and Hold : dspsigops/Sample and Hold  trig=Rising edge  initCond=0  latchinput=on
  E-Lin : Outport
  wires:
  Velocity MF/1 -> Product/1
  Force Impedance Delayed/1 -> Product/2
  Product/1 -> Add/2
  Sample and Hold/1 -> Add/1
  Add/1 -> Sample and Hold/1, E-Lin/1
  Clock/1 -> Sample and Hold/Trigger

== system NUOVO_MODELLO_COPPIE_VELOCITA/POPC - Slave Side2/PASSIVE OBSERVER Right Output ==
  Force Impedence : Inport
  Velocity Slave : Inport  Port=2
  Add : Sum
  Clock : simulink_extras/Flip Flops/Clock  period=Ts*2
  Product : Product
  Sample and Hold : dspsigops/Sample and Hold  trig=Rising edge  initCond=0  latchinput=on
  E-Rout : Outport
  wires:
  Velocity Slave/1 -> Product/1
  Force Impedence/1 -> Product/2
  Product/1 -> Add/2
  Sample and Hold/1 -> Add/1
  Add/1 -> Sample and Hold/1, E-Rout/1
  Clock/1 -> Sample and Hold/Trigger

== system NUOVO_MODELLO_COPPIE_VELOCITA/POPC - Slave Side2/PC Slave ==
  Energy POs : Inport
  Velocity Slave : Inport  Port=2
  Clock1 : simulink_extras/Flip Flops/Clock  period=Ts*2
  PASSIVE CONTROLLER PCs : MATLAB Function  TreatAsAtomicUnit=on
  Sample and Hold1 : dspsigops/Sample and Hold  trig=Rising edge  initCond=0  latchinput=on
  dt1 : Constant  Value=dt
  Energy PC : Outport
  ALPHA : Outport  Port=2
  wires:
  PASSIVE CONTROLLER PCs/1(E_PCs) -> Sample and Hold1/1
  dt1/1 -> PASSIVE CONTROLLER PCs/3(Ts)
  PASSIVE CONTROLLER PCs/2(alpha_s) -> ALPHA/1
  Energy POs/1 -> PASSIVE CONTROLLER PCs/2(E_POs)
  Clock1/1 -> Sample and Hold1/Trigger
  Sample and Hold1/1 -> Energy PC/1, PASSIVE CONTROLLER PCs/1(E_PCs_prev)
  Velocity Slave/1 -> PASSIVE CONTROLLER PCs/4(v_s)

== system NUOVO_MODELLO_COPPIE_VELOCITA/SLAVE_SIDE 2/Environment  ==
  Pos_Slave : Inport
  "Vel_Slave " : Inport  Port=2
  Environment Behaviour : MATLAB Function  TreatAsAtomicUnit=on
  Environment Position : Constant  Value=qe
  Stiffness : Constant  Value=Ke
  Viscous Friction : Constant  Value=Be
  Fe : Outport
  wires:
  Pos_Slave/1 -> Environment Behaviour/1(x_s)
  "Vel_Slave "/1 -> Environment Behaviour/2(dot_x_s)
  Environment Position/1 -> Environment Behaviour/3(qe)
  Viscous Friction/1 -> Environment Behaviour/4(Be)
  Stiffness/1 -> Environment Behaviour/5(Ke)
  Environment Behaviour/1(Fe) -> Fe/1

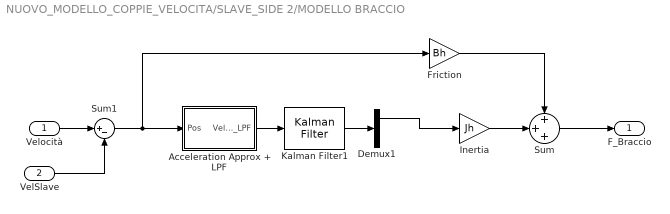
== system NUOVO_MODELLO_COPPIE_VELOCITA/SLAVE_SIDE 2/MODELLO BRACCIO ==
  "Velocità " : Inport
  VelSlave : Inport  Port=2
  "Acceleration Approx + LPF " : Subsystem
  Demux1 : Demux  Outputs=2
  Friction : Gain  Gain=Bh
  Inertia : Gain  Gain=Jh
  Kalman Filter1 : ctrlSharedLib/Kalman Filter  TimeDomain=Discrete-Time  UseCurrentEstimator=off  ModelSource=Individual A, B, C, D matrices  ModelSourceVariable=ss(A,0,C,0)  A=A  B=1  C=C  D=0  NumberOfStates=2  NumberOfInputs=1  NumberOfOutputs=1  InitialEstimateSource=Dialog  X0=0  P0=10  UseK=off  UseGH=off  NumberOfProcessNoiseInputs=1  G=1  TimeInvariantG=on  H=0  TimeInvariantH=on  Q=0.05  TimeInvariantQ=on  R=1  TimeInvariantR=on  N=0  TimeInvariantN=on  AddInputPort=off  AddEnablePort=off  OutputEstimatedY=off  OutputP=off  Ts=Ts
  Sum : Sum  Inputs=+++
  Sum1 : Sum  Inputs=|+-
  F_Braccio : Outport
  wires:
  Sum1/1 -> "Acceleration Approx + LPF "/1(Pos), Friction/1
  Inertia/1 -> Sum/2
  Friction/1 -> Sum/1
  Sum/1 -> F_Braccio/1
  "Acceleration Approx + LPF "/1("Vel_H_LPF ") -> Kalman Filter1/1
  Kalman Filter1/1 -> Demux1/1
  Demux1/1 -> Inertia/1
  "Velocità "/1 -> Sum1/1
  VelSlave/1 -> Sum1/2

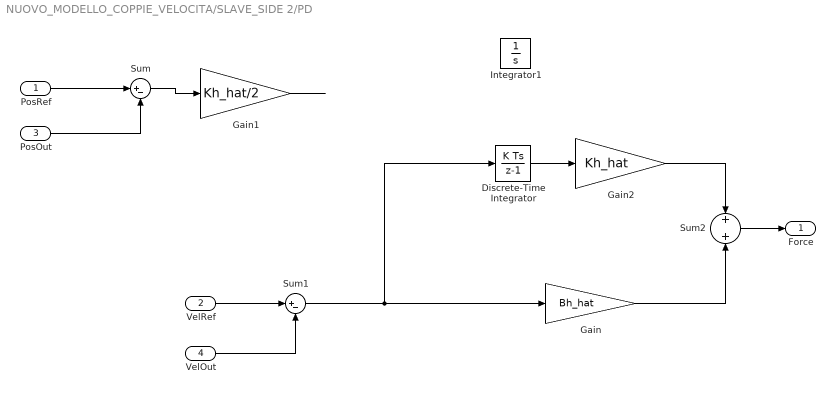
== system NUOVO_MODELLO_COPPIE_VELOCITA/SLAVE_SIDE 2/PD ==
  PosRef : Inport
  VelRef : Inport  Port=2
  PosOut : Inport  Port=3
  VelOut : Inport  Port=4
  Discrete-Time Integrator : DiscreteIntegrator  SampleTime=-1  ICPrevOutput=DiscIntNeverNeededParam  ICPrevScaledInput=DiscIntNeverNeededParam
  Gain : Gain  Gain=Bh_hat
  Gain1 : Gain  Gain=Kh_hat/2
  Gain2 : Gain  Gain=Kh_hat
  Integrator1 : Integrator
  Sum : Sum  Inputs=|+-
  Sum1 : Sum  Inputs=|+-
  Sum2 : Sum
  Force : Outport
  wires:
  PosRef/1 -> Sum/1
  PosOut/1 -> Sum/2
  VelRef/1 -> Sum1/1
  VelOut/1 -> Sum1/2
  Sum1/1 -> Discrete-Time Integrator/1, Gain/1
  Sum/1 -> Gain1/1
  Gain1/1 -> ?
  Gain/1 -> Sum2/2
  Sum2/1 -> Force/1
  Discrete-Time Integrator/1 -> Gain2/1
  Gain2/1 -> Sum2/1

== system NUOVO_MODELLO_COPPIE_VELOCITA/SLAVE_SIDE 2/Velocity Approx + LPF  ==
  Pos : Inport
  Clock : simulink_extras/Flip Flops/Clock  period=Ts*2
  Clock1 : simulink_extras/Flip Flops/Clock  period=Ts*2
  Constant : Constant  Value=Ts
  Constant1 : Constant  Value=beta
  "Euler Approximation " : MATLAB Function  TreatAsAtomicUnit=on
  Sample and Hold : dspsigops/Sample and Hold  trig=Rising edge  initCond=0  latchinput=on
  Sample and Hold1 : dspsigops/Sample and Hold  trig=Rising edge  initCond=0  latchinput=on
  "Vel_H_LPF " : Outport
  wires:
  Pos/1 -> Sample and Hold/1, "Euler Approximation "/3(pos)
  Constant/1 -> "Euler Approximation "/2(Ts)
  Sample and Hold/1 -> "Euler Approximation "/4(posPrev)
  Clock/1 -> Sample and Hold/Trigger
  Sample and Hold1/1 -> "Euler Approximation "/5(filteredPrev)
  "Euler Approximation "/1(filtered) -> "Vel_H_LPF "/1, Sample and Hold1/1
  Clock1/1 -> Sample and Hold1/Trigger
  Constant1/1 -> "Euler Approximation "/1(beta)

== system NUOVO_MODELLO_COPPIE_VELOCITA/POPC - Master Side2/PO Input - Slave to Master (Cause)/PASSIVE OBSERVER S2M E Right INPUT ==
  Env_Force : Inport
  "Vel_M " : Inport  Port=2
  Clock : simulink_extras/Flip Flops/Clock  period=Ts*2
  Product : Product
  Sample and Hold : dspsigops/Sample and Hold  trig=Rising edge  initCond=0  latchinput=on
  Sum : Sum
  E-Rin : Outport
  wires:
  Env_Force/1 -> Product/1
  "Vel_M "/1 -> Product/2
  Product/1 -> Sum/2
  Sum/1 -> Sample and Hold/1, E-Rin/1
  Sample and Hold/1 -> Sum/1
  Clock/1 -> Sample and Hold/Trigger

== system NUOVO_MODELLO_COPPIE_VELOCITA/POPC - Master Side2/PO Output - Master to Slave (Effect)/PASSIVE OBSERVER M2S E Left OUTPUT ==
  Velocity Master : Inport
  Force Env Delayed : Inport  Port=2
  Clock : simulink_extras/Flip Flops/Clock  period=Ts*2
  Product : Product
  Sample and Hold : dspsigops/Sample and Hold  trig=Rising edge  initCond=0  latchinput=on
  Sum : Sum
  E-Lout : Outport
  wires:
  Velocity Master/1 -> Product/1
  Force Env Delayed/1 -> Product/2
  Product/1 -> Sum/2
  Sample and Hold/1 -> Sum/1
  Sum/1 -> Sample and Hold/1, E-Lout/1
  Clock/1 -> Sample and Hold/Trigger

== system NUOVO_MODELLO_COPPIE_VELOCITA/SLAVE_SIDE 2/MODELLO BRACCIO/Acceleration Approx + LPF  ==
  Pos : Inport
  Clock : simulink_extras/Flip Flops/Clock  period=Ts*2
  Clock1 : simulink_extras/Flip Flops/Clock  period=Ts*2
  Constant : Constant  Value=Ts
  Constant1 : Constant  Value=beta
  "Euler Approximation " : MATLAB Function  TreatAsAtomicUnit=on
  Sample and Hold : dspsigops/Sample and Hold  trig=Rising edge  initCond=0  latchinput=on
  Sample and Hold1 : dspsigops/Sample and Hold  trig=Rising edge  initCond=0  latchinput=on
  "Vel_H_LPF " : Outport
  wires:
  Pos/1 -> Sample and Hold/1, "Euler Approximation "/3(pos)
  Constant/1 -> "Euler Approximation "/2(Ts)
  Sample and Hold/1 -> "Euler Approximation "/4(posPrev)
  Clock/1 -> Sample and Hold/Trigger
  Sample and Hold1/1 -> "Euler Approximation "/5(filteredPrev)
  "Euler Approximation "/1(filtered) -> "Vel_H_LPF "/1, Sample and Hold1/1
  Clock1/1 -> Sample and Hold1/Trigger
  Constant1/1 -> "Euler Approximation "/1(beta)

== matlab function NUOVO_MODELLO_COPPIE_VELOCITA/POPC - Slave Side2/PC Slave/PASSIVE CONTROLLER PCs ==
  data: E_PCs_prev input; E_POs input; E_PCs output; Ts input; v_s input; alpha_s output
function [E_PCs, alpha_s]= PC_s(E_PCs_prev, E_POs, Ts, v_s)

if (E_POs < 0 && v_s ~= 0)
    alpha_s = (-E_POs)/Ts*v_s^2;
else
    alpha_s = 0;
end

E_PCs = E_PCs_prev + (alpha_s*v_s^2)*Ts;

== matlab function NUOVO_MODELLO_COPPIE_VELOCITA/SLAVE_SIDE 2/Environment /Environment Behaviour ==
  data: x_s input; Fe output; dot_x_s input; qe input; Be input; Ke input
function Fe = Env(x_s, dot_x_s, qe, Be, Ke)
    
    if(x_s > qe)
        Fe = Ke*(x_s - qe) + Be*dot_x_s;
    else
        Fe = 0;
    end

== matlab function NUOVO_MODELLO_COPPIE_VELOCITA/MASTER SIDE/Noise Gate ==
  data: u input; y output; noise_threshold input
function y = noise_gate(u, noise_threshold)

if(u <= -noise_threshold || u >= noise_threshold)
    y = u;
else
    y = 0;
end

== matlab function NUOVO_MODELLO_COPPIE_VELOCITA/SLAVE_SIDE 2/Velocity Approx + LPF /Euler Approximation  ==
  data: beta input; Ts input; filtered output; pos input; posPrev input; filteredPrev input
function filtered = EulApprox(beta, Ts, pos, posPrev, filteredPrev)

eul= (pos - posPrev)/Ts;
filtered = beta*eul + (1-beta)*filteredPrev;

== matlab function NUOVO_MODELLO_COPPIE_VELOCITA/SLAVE_SIDE 2/MODELLO BRACCIO/Acceleration Approx + LPF /Euler Approximation  ==
  data: beta input; Ts input; filtered output; pos input; posPrev input; filteredPrev input
function filtered = EulApprox(beta, Ts, pos, posPrev, filteredPrev)

eul= (pos - posPrev)/Ts;
filtered = beta*eul + (1-beta)*filteredPrev;

== matlab function NUOVO_MODELLO_COPPIE_VELOCITA/MASTER SIDE/Velocity Approx + LPF 6/Euler Approximation  ==
  data: beta input; Ts input; filtered output; pos input; posPrev input; filteredPrev input
function filtered = EulApprox(beta, Ts, pos, posPrev, filteredPrev)

eul= (pos - posPrev)/Ts;
filtered = beta*eul + (1-beta)*filteredPrev;

== matlab function NUOVO_MODELLO_COPPIE_VELOCITA/Euler Approximation Vel M2/Euler Approximation  ==
  data: beta input; Ts input; filtered output; pos input; posPrev input; filteredPrev input
function filtered = EulApprox(beta, Ts, pos, posPrev, filteredPrev)

eul= (pos - posPrev)/Ts;
filtered = beta*eul + (1-beta)*filteredPrev;

== matlab function NUOVO_MODELLO_COPPIE_VELOCITA/MASTER SIDE/Velocity Approx + LPF /Euler Approximation  ==
  data: beta input; Ts input; filtered output; pos input; posPrev input; filteredPrev input
function filtered = EulApprox(beta, Ts, pos, posPrev, filteredPrev)

eul= (pos - posPrev)/Ts;
filtered = beta*eul + (1-beta)*filteredPrev;

== matlab function NUOVO_MODELLO_COPPIE_VELOCITA/MASTER SIDE/Velocity Approx + LPF 1/Euler Approximation  ==
  data: beta input; Ts input; filtered output; pos input; posPrev input; filteredPrev input
function filtered = EulApprox(beta, Ts, pos, posPrev, filteredPrev)

eul= (pos - posPrev)/Ts;
filtered = beta*eul + (1-beta)*filteredPrev;

== matlab function NUOVO_MODELLO_COPPIE_VELOCITA/MASTER SIDE/Velocity Approx + LPF 2/Euler Approximation  ==
  data: beta input; Ts input; filtered output; pos input; posPrev input; filteredPrev input
function filtered = EulApprox(beta, Ts, pos, posPrev, filteredPrev)

eul= (pos - posPrev)/Ts;
filtered = beta*eul + (1-beta)*filteredPrev;

== matlab function NUOVO_MODELLO_COPPIE_VELOCITA/Operator Stiffness2/Operator Stiffness  ==
  data: KhMax input; Kh input; Kh_func output; t input; stopTime input
function Kh_func = stiffness(KhMax, Kh, t, stopTime)
%Solving cubic polynomial function to model the operator stiffness
%(f'(begin) + f'(end) - 2*f(begin))(x/k)^3 + (3*f(end) - 2*f'(begin) - f'(end))(x/k)^2 + f'(begin)x/k + f(begin)

    begin = 0.5;

    endTime = stopTime-0.5;

    df_begin = 0;
    df_end = 0;
    f_end = KhMax - Kh;

    if t < begin
    Kh_func = Kh;
    else
    Kh_func = (df_begin + df_end - 2*f_end)*((t-begin)/endTime)^3 + (3*f_end - 2*df_begin - df_end)*((t-begin)/endTime)^2 + (df_begin)*((t-begin)/endTime) + Kh;
    end
end

== matlab function NUOVO_MODELLO_COPPIE_VELOCITA/POPC - Master Side2/PC - Master side/PASSIVE CONTROLLER PCm ==
  data: E_POm input; E_PCm output; dt input; v_m input; E_PCm_prev input; alpha_m output
function [E_PCm, alpha_m]= PC_m(E_POm, dt, v_m, E_PCm_prev)

if (E_POm < 0 && v_m ~= 0)
    alpha_m = (-E_POm)/dt*v_m^2;
else
    alpha_m = 0;
end

E_PCm = E_PCm_prev + (alpha_m*v_m^2)*dt;
